simulink model "LCC_TrajectoryPlanning"  (R2025b)
settings: Solver=FixedStepDiscrete  StartTime=0.0  StopTime=10  FixedStep=.05  RelTol=1e-3
libraries: simulink_extras x1
settings Model: PacingRate=0.500000  Creator=scb548  LastModifiedBy=Sam Ball
settings OptimizationCC: ZeroExternalMemoryAtStartup=off  ZeroInternalMemoryAtStartup=off
settings RTWCC: SystemTargetFile=rtmaps.tlc  TemplateMakefile=rtmaps_default_tmf  PostCodeGenCommand=rtmaps_post_code_generation(buildInfo)  RetainRTWFile=on  TargetLang=C++  GPUComputeCapability=3.5  Description=Generate an RTMaps component embedding the model
settings STFCustomTargetCC: SystemTargetFile=rtmaps.tlc  TargetLangStandard=C++11 (ISO)  ModelReferenceCompliant=off  CombineOutputUpdateFcns=on  CodeInterfacePackaging=C++ class  SubcomponentCodeInterfacePackaging=C++ class  CPPClassGenCompliant=on  GRTInterface=off  RTMAPS_SDKDIR=/opt/rtmaps  RTMAPS_BOARD=ubuntu2204_x86_64  DisplayOptimOptions=off  RTMaps_MatFileLogging=0  CustomFileTemplate=rtmaps_file_process.tlc  RTMaps_GRTInterface=0  RTMaps_GenerateERTSFunction=0  RTMaps_IntegerCode=0  RTMaps_GenerateAllocFcn=0  RTMAPS_OS=ubuntu2204  RTMaps_CombineOutputUpdateFcns=1  RTMaps_MultiInstanceCode=1  RTMAPS_ARCH=x86_64
settings GRTTargetCC: TargetLangStandard=C++11 (ISO)  ModelReferenceCompliant=off  ParMdlRefBuildCompliant=off  CompOptLevelCompliant=off  MatFileLogging=off  CodeInterfacePackaging=C++ class  SubcomponentCodeInterfacePackaging=C++ class  UseToolchainInfoCompliant=off

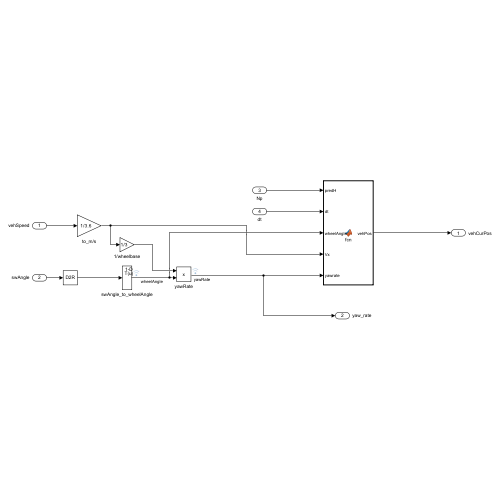
[thumbnail: Simulink's stored preview of the top-level diagram]
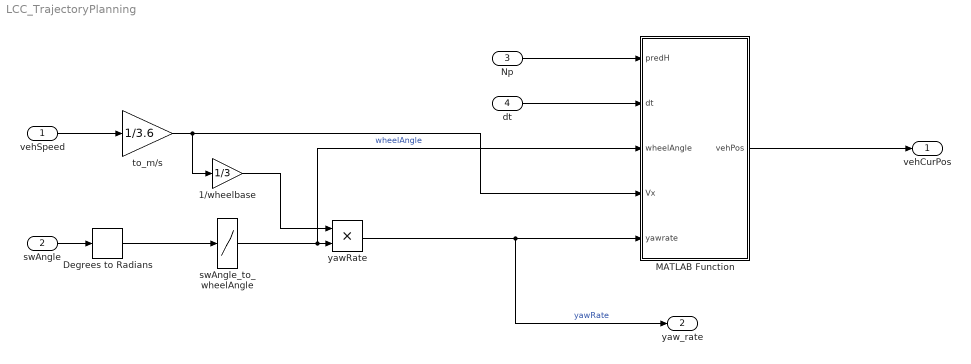
== system LCC_TrajectoryPlanning ==
  vehSpeed : Inport
  swAngle : Inport  Port=2
  Np : Inport  Port=3
  dt : Inport  Port=4
  1/wheelbase : Gain  Gain=1/3
  Degrees to Radians : simulink_extras/Transformations/Degrees to Radians
  MATLAB Function : MATLAB Function  TreatAsAtomicUnit=on
  swAngle_to_wheelAngle : Lookup_n-D  NumberOfTableDimensions=1  BreakpointsForDimension1=[-10.89089966;-10.16600037;-9.441100121;-8.716199875;-7.991300106;-7.26639986;-6.541500092;-5.816599846;-5.091700077;-4.366799831;-3.641900063;-2.917000055;-2.192100048;-1.467200041;-0.742299974;-0.0175;0.0175;0.742299974;1.467200041;2.192100048;2.917000055;3.641900063;4.366799831;5.091700077;5.816599846;6.541500092;7.26639986;7.991300106;8.716199875;9.441100121;10.16600037;10.89089966]  Table=[-0.636900008;-0.589100003;-0.539099991;-0.490500003;-0.44659999;-0.404900014;-0.361499995;-0.317299992;-0.27610001;-0.237499997;-0.197899997;-0.156399995;-0.1162;-0.078699999;-0.041099999;-0.001;0.001;0.041200001;0.079099998;0.116499998;0.156399995;0.197999999;0.237900004;0.276499987;0.317400008;0.361499995;0.405299991;0.447100013;0.490700006;0.539099991;0.589399993;0.637499988]  InternalRulePriority=Speed  RndMeth=Simplest
  to_m/s : Gain  Gain=1/3.6
  yawRate : Product
  vehCurPos : Outport
  yaw_rate : Outport  Port=2
  wires:
  swAngle/1 -> Degrees to Radians/1
  vehSpeed/1 -> to_m/s/1
  Degrees to Radians/1 -> swAngle_to_wheelAngle/1
  to_m/s/1 -> MATLAB Function/4(Vx), 1/wheelbase/1
  1/wheelbase/1 -> yawRate/1
  swAngle_to_wheelAngle/1 -> MATLAB Function/3(wheelAngle), yawRate/2  "wheelAngle"
  yawRate/1 -> MATLAB Function/5(yawrate), yaw_rate/1  "yawRate"
  Np/1 -> MATLAB Function/1(predH)
  dt/1 -> MATLAB Function/2(dt)
  MATLAB Function/1(vehPos) -> vehCurPos/1

== matlab function LCC_TrajectoryPlanning/MATLAB Function ==
  data: predH input; vehPos output; dt input; wheelAngle input; Vx input; yawrate input
function vehPos = fcn(predH, dt, wheelAngle, Vx, yawrate)

% Vehicle parameters
m = 2721.6;
Jz = 2624;
lf = 1.5;
lr = 1.5;
Cf = 12000;
Cr = 20000;
Vx = max(Vx, 0.1);

x = [Vx*sin(wheelAngle); yawrate; wheelAngle; 0]; % vy, yawrate, yaw, y
u = wheelAngle;

position = zeros(predH,2);
        
% Continuous model
A = [-(Cf+Cr)/(m*Vx), -Vx - (Cf*lf - Cr*lr)/(m*Vx), 0, 0;
     -(Cf*lf - Cr*lr)/(Jz*Vx), -(Cf*lf^2 + Cr*lr^2)/(Jz*Vx), 0, 0;
     0, 1, 0, 0;
     1, 0, Vx, 0];
B = [Cf/m; (Cf*lf)/Jz; 0; 0];
C = [0 0 1 0; 0 0 0 1]; % Extract yaw and lateral position

% Discrete Model
Ad = eye(4) + A*dt;
Bd = B*dt*10;

for i = 1:predH

    x = Ad*x + Bd*u;
    position(i, :) = (C*x).'; % yaw and lateral position

end

vehPos = position(5,:);
